simulink model "case8"  (R2024b)
settings: Solver=FixedStepAuto  StartTime=0  StopTime=1  FixedStep=1e-7  RelTol=1e-3
values from neighbouring files (symbols this model uses):
  SG_D_1_D = 0.01056    [IEEE9_case_parameters.m]    (also in case1_parameters.m; case2_parameters.m; case3_parameters.m; case4_parameters.m)
  SG_D_1_EnableSaturation = 0    [IEEE9_case_parameters.m]    (also in case1_parameters.m; case2_parameters.m; case3_parameters.m; case4_parameters.m)
  SG_D_1_f0 = 60    [IEEE9_case_parameters.m]    (also in case1_parameters.m; case2_parameters.m; case3_parameters.m; case4_parameters.m)
  SG_D_1_H = 7.5    [IEEE9_case_parameters.m]    (also in case1_parameters.m; case2_parameters.m; case3_parameters.m; case4_parameters.m)
  SG_D_1_K_A = 20    [IEEE9_case_parameters.m]    (also in case1_parameters.m; case2_parameters.m; case3_parameters.m; case4_parameters.m)
  SG_D_1_K_E = 1.000000e+1    (= 10)    [IEEE9_case_parameters.m]    (also in case1_parameters.m; case2_parameters.m; case3_parameters.m; case4_parameters.m)
  SG_D_1_K_F = 2.363    [IEEE9_case_parameters.m]    (also in case1_parameters.m; case2_parameters.m; case3_parameters.m; case4_parameters.m)
  SG_D_1_K_s = 0.5    [IEEE9_case_parameters.m]    (also in case1_parameters.m = 5; case2_parameters.m = 5; case3_parameters.m = 5; case4_parameters.m = 5)
  SG_D_1_R_a = 0.001088    [IEEE9_case_parameters.m]    (also in case1_parameters.m; case2_parameters.m; case3_parameters.m; case4_parameters.m)
  SG_D_1_S_A = 1    [IEEE9_case_parameters.m]    (also in case1_parameters.m; case2_parameters.m; case3_parameters.m; case4_parameters.m)
  SG_D_1_S_B = 0.103    [IEEE9_case_parameters.m]    (also in case1_parameters.m; case2_parameters.m; case3_parameters.m; case4_parameters.m)
  SG_D_1_S_N = 10.659857    [IEEE9_case_parameters.m]    (also in case1_parameters.m; case2_parameters.m; case3_parameters.m; case4_parameters.m)
  SG_D_1_SpeedPara = 200    [IEEE9_case_parameters.m]    (also in case1_parameters.m; case2_parameters.m; case3_parameters.m; case4_parameters.m)
  SG_D_1_T_0 = 0.720173    [IEEE9_case_parameters.m]    (also in case1_parameters.m = 0.755522; case2_parameters.m = 0.808931; case3_parameters.m = 0.869402; case4_parameters.m = 0.729316)
  SG_D_1_T_1 = 0.3    [IEEE9_case_parameters.m]    (also in case1_parameters.m; case2_parameters.m; case3_parameters.m; case4_parameters.m)
  SG_D_1_T_2 = 0.05    [IEEE9_case_parameters.m]    (also in case1_parameters.m; case2_parameters.m; case3_parameters.m; case4_parameters.m)
  SG_D_1_T_3 = 0.02    [IEEE9_case_parameters.m]    (also in case1_parameters.m; case2_parameters.m; case3_parameters.m; case4_parameters.m)
  SG_D_1_T_4 = 0.005    [IEEE9_case_parameters.m]    (also in case1_parameters.m; case2_parameters.m; case3_parameters.m; case4_parameters.m)
  SG_D_1_T_A = 0.02    [IEEE9_case_parameters.m]    (also in case1_parameters.m; case2_parameters.m; case3_parameters.m; case4_parameters.m)
  SG_D_1_T_dd = 8.000000e+0    (= 8)    [IEEE9_case_parameters.m]    (also in case1_parameters.m; case2_parameters.m; case3_parameters.m; case4_parameters.m)
  SG_D_1_T_ddd = 0.04    [IEEE9_case_parameters.m]    (also in case1_parameters.m; case2_parameters.m; case3_parameters.m; case4_parameters.m)
  SG_D_1_T_E = 0.314    [IEEE9_case_parameters.m]    (also in case1_parameters.m; case2_parameters.m; case3_parameters.m; case4_parameters.m)
  SG_D_1_T_F = 0.35    [IEEE9_case_parameters.m]    (also in case1_parameters.m; case2_parameters.m; case3_parameters.m; case4_parameters.m)
  SG_D_1_T_qd = 0.8    [IEEE9_case_parameters.m]    (also in case1_parameters.m; case2_parameters.m; case3_parameters.m; case4_parameters.m)
  SG_D_1_T_qdd = 0.02    [IEEE9_case_parameters.m]    (also in case1_parameters.m; case2_parameters.m; case3_parameters.m; case4_parameters.m)
  SG_D_1_T_speed = 0.1    [IEEE9_case_parameters.m]    (also in case1_parameters.m = 200; case2_parameters.m = 200; case3_parameters.m = 200; case4_parameters.m = 200)
  SG_D_1_T_w = 0.5    [IEEE9_case_parameters.m]    (also in case1_parameters.m; case2_parameters.m; case3_parameters.m; case4_parameters.m)
  SG_D_1_V_ref = 1.990276    [IEEE9_case_parameters.m]    (also in case1_parameters.m = 2.042296; case2_parameters.m = 2.051388; case3_parameters.m = 2.089584; case4_parameters.m = 2.01845)
  SG_D_1_w_ref = 376.991118    [IEEE9_case_parameters.m]    (also in case1_parameters.m; case2_parameters.m; case3_parameters.m; case4_parameters.m)
  SG_D_1_wb = 6.000000e+1    (= 60)    [IEEE9_case_parameters.m]    (also in case1_parameters.m; case2_parameters.m; case3_parameters.m; case4_parameters.m)
  SG_D_1_x_d = 1.9    [IEEE9_case_parameters.m]    (also in case1_parameters.m; case2_parameters.m; case3_parameters.m; case4_parameters.m)
  SG_D_1_x_dd = 0.302    [IEEE9_case_parameters.m]    (also in case1_parameters.m; case2_parameters.m; case3_parameters.m; case4_parameters.m)
  SG_D_1_x_ddd = 0.204    [IEEE9_case_parameters.m]    (also in case1_parameters.m; case2_parameters.m; case3_parameters.m; case4_parameters.m)
  SG_D_1_x_l = 0.05    [IEEE9_case_parameters.m]    (also in case1_parameters.m; case2_parameters.m; case3_parameters.m; case4_parameters.m)
  SG_D_1_x_q = 1.3    [IEEE9_case_parameters.m]    (also in case1_parameters.m; case2_parameters.m; case3_parameters.m; case4_parameters.m)
  SG_D_1_x_qd = 0.5    [IEEE9_case_parameters.m]    (also in case1_parameters.m; case2_parameters.m; case3_parameters.m; case4_parameters.m)
  SG_D_1_x_qdd = 0.3    [IEEE9_case_parameters.m]    (also in case1_parameters.m; case2_parameters.m; case3_parameters.m; case4_parameters.m)
  SG_D_2_D = 0.02    [IEEE9_case_parameters.m]    (also in case1_parameters.m; case2_parameters.m; case3_parameters.m; case4_parameters.m)
  SG_D_2_EnableSaturation = 0    [IEEE9_case_parameters.m]    (also in case1_parameters.m; case2_parameters.m; case3_parameters.m; case4_parameters.m)
  SG_D_2_f0 = 60    [IEEE9_case_parameters.m]    (also in case1_parameters.m; case2_parameters.m; case3_parameters.m; case4_parameters.m)
  SG_D_2_H = 8.000000e+0    (= 8)    [IEEE9_case_parameters.m]    (also in case1_parameters.m; case2_parameters.m; case3_parameters.m; case4_parameters.m)
  SG_D_2_K_A = 20    [IEEE9_case_parameters.m]    (also in case1_parameters.m; case2_parameters.m; case3_parameters.m; case4_parameters.m)
  SG_D_2_K_E = 1.000000e+1    (= 10)    [IEEE9_case_parameters.m]    (also in case1_parameters.m; case2_parameters.m; case3_parameters.m; case4_parameters.m)
  SG_D_2_K_F = 2.363    [IEEE9_case_parameters.m]    (also in case1_parameters.m; case2_parameters.m; case3_parameters.m; case4_parameters.m)
  SG_D_2_K_s = 0.5    [IEEE9_case_parameters.m]    (also in case1_parameters.m = 4; case2_parameters.m = 4; case3_parameters.m = 4; case4_parameters.m = 4)
  SG_D_2_R_a = 0.001088    [IEEE9_case_parameters.m]    (also in case1_parameters.m; case2_parameters.m; case3_parameters.m; case4_parameters.m)
  SG_D_2_S_A = 1    [IEEE9_case_parameters.m]    (also in case1_parameters.m; case2_parameters.m; case3_parameters.m; case4_parameters.m)
  SG_D_2_S_B = 0.103    [IEEE9_case_parameters.m]    (also in case1_parameters.m; case2_parameters.m; case3_parameters.m; case4_parameters.m)
  SG_D_2_S_N = 10.659857    [IEEE9_case_parameters.m]    (also in case1_parameters.m; case2_parameters.m; case3_parameters.m; case4_parameters.m)
  SG_D_2_SpeedPara = 200    [IEEE9_case_parameters.m]    (also in case1_parameters.m; case2_parameters.m; case3_parameters.m; case4_parameters.m)
  SG_D_2_T_0 = 1.632913    [IEEE9_case_parameters.m]    (also in case1_parameters.m = 1.632925; case2_parameters.m = 1.632915; case3_parameters.m = 1.632914; case4_parameters.m = 1.632927)
  SG_D_2_T_1 = 0.2    [IEEE9_case_parameters.m]    (also in case1_parameters.m; case2_parameters.m; case3_parameters.m; case4_parameters.m)
  SG_D_2_T_2 = 0.05    [IEEE9_case_parameters.m]    (also in case1_parameters.m; case2_parameters.m; case3_parameters.m; case4_parameters.m)
  SG_D_2_T_3 = 0.02    [IEEE9_case_parameters.m]    (also in case1_parameters.m; case2_parameters.m; case3_parameters.m; case4_parameters.m)
  SG_D_2_T_4 = 0.005    [IEEE9_case_parameters.m]    (also in case1_parameters.m; case2_parameters.m; case3_parameters.m; case4_parameters.m)
  SG_D_2_T_A = 0.02    [IEEE9_case_parameters.m]    (also in case1_parameters.m; case2_parameters.m; case3_parameters.m; case4_parameters.m)
  SG_D_2_T_dd = 7.9    [IEEE9_case_parameters.m]    (also in case1_parameters.m; case2_parameters.m; case3_parameters.m; case4_parameters.m)
  SG_D_2_T_ddd = 0.04    [IEEE9_case_parameters.m]    (also in case1_parameters.m; case2_parameters.m; case3_parameters.m; case4_parameters.m)
  SG_D_2_T_E = 0.314    [IEEE9_case_parameters.m]    (also in case1_parameters.m; case2_parameters.m; case3_parameters.m; case4_parameters.m)
  SG_D_2_T_F = 0.35    [IEEE9_case_parameters.m]    (also in case1_parameters.m; case2_parameters.m; case3_parameters.m; case4_parameters.m)
  SG_D_2_T_qd = 0.8    [IEEE9_case_parameters.m]    (also in case1_parameters.m; case2_parameters.m; case3_parameters.m; case4_parameters.m)
  SG_D_2_T_qdd = 0.015    [IEEE9_case_parameters.m]    (also in case1_parameters.m; case2_parameters.m; case3_parameters.m; case4_parameters.m)
  SG_D_2_T_speed = 0.1    [IEEE9_case_parameters.m]    (also in case1_parameters.m = 150; case2_parameters.m = 150; case3_parameters.m = 150; case4_parameters.m = 150)
  SG_D_2_T_w = 0.35    [IEEE9_case_parameters.m]    (also in case1_parameters.m; case2_parameters.m; case3_parameters.m; case4_parameters.m)
  SG_D_2_V_ref = 2.58547    [IEEE9_case_parameters.m]    (also in case1_parameters.m = 2.597896; case2_parameters.m = 2.587136; case3_parameters.m = 2.586042; case4_parameters.m = 2.599679)
  SG_D_2_w_ref = 376.991118    [IEEE9_case_parameters.m]    (also in case1_parameters.m; case2_parameters.m; case3_parameters.m; case4_parameters.m)
  SG_D_2_wb = 6.000000e+1    (= 60)    [IEEE9_case_parameters.m]    (also in case1_parameters.m; case2_parameters.m; case3_parameters.m; case4_parameters.m)
  SG_D_2_x_d = 1.8    [IEEE9_case_parameters.m]    (also in case1_parameters.m; case2_parameters.m; case3_parameters.m; case4_parameters.m)
  SG_D_2_x_dd = 0.302    [IEEE9_case_parameters.m]    (also in case1_parameters.m; case2_parameters.m; case3_parameters.m; case4_parameters.m)
  SG_D_2_x_ddd = 0.204    [IEEE9_case_parameters.m]    (also in case1_parameters.m; case2_parameters.m; case3_parameters.m; case4_parameters.m)
  SG_D_2_x_l = 0.05    [IEEE9_case_parameters.m]    (also in case1_parameters.m; case2_parameters.m; case3_parameters.m; case4_parameters.m)
  SG_D_2_x_q = 1.25    [IEEE9_case_parameters.m]    (also in case1_parameters.m; case2_parameters.m; case3_parameters.m; case4_parameters.m)
  SG_D_2_x_qd = 0.5    [IEEE9_case_parameters.m]    (also in case1_parameters.m; case2_parameters.m; case3_parameters.m; case4_parameters.m)
  SG_D_2_x_qdd = 0.3    [IEEE9_case_parameters.m]    (also in case1_parameters.m; case2_parameters.m; case3_parameters.m; case4_parameters.m)
  SG_D_3_D = 0.02    [IEEE9_case_parameters.m]    (also in case1_parameters.m; case2_parameters.m; case3_parameters.m; case4_parameters.m)
  SG_D_3_EnableSaturation = 0    [IEEE9_case_parameters.m]    (also in case1_parameters.m; case2_parameters.m; case3_parameters.m; case4_parameters.m)
  SG_D_3_f0 = 60    [IEEE9_case_parameters.m]    (also in case1_parameters.m; case2_parameters.m; case3_parameters.m; case4_parameters.m)
  SG_D_3_H = 7.7    [IEEE9_case_parameters.m]    (also in case1_parameters.m; case2_parameters.m; case3_parameters.m; case4_parameters.m)
  SG_D_3_K_A = 20    [IEEE9_case_parameters.m]    (also in case1_parameters.m; case2_parameters.m; case3_parameters.m; case4_parameters.m)
  SG_D_3_K_E = 1.000000e+1    (= 10)    [IEEE9_case_parameters.m]    (also in case1_parameters.m; case2_parameters.m; case3_parameters.m; case4_parameters.m)
  SG_D_3_K_F = 2.363    [IEEE9_case_parameters.m]    (also in case1_parameters.m; case2_parameters.m; case3_parameters.m; case4_parameters.m)
  SG_D_3_K_s = 0.2    [IEEE9_case_parameters.m]    (also in case1_parameters.m = 2; case2_parameters.m = 2; case3_parameters.m = 2; case4_parameters.m = 2)
  SG_D_3_R_a = 0.001088    [IEEE9_case_parameters.m]    (also in case1_parameters.m; case2_parameters.m; case3_parameters.m; case4_parameters.m)
  SG_D_3_S_A = 1    [IEEE9_case_parameters.m]    (also in case1_parameters.m; case2_parameters.m; case3_parameters.m; case4_parameters.m)
  SG_D_3_S_B = 0.103    [IEEE9_case_parameters.m]    (also in case1_parameters.m; case2_parameters.m; case3_parameters.m; case4_parameters.m)
  SG_D_3_S_N = 10.659857    [IEEE9_case_parameters.m]    (also in case1_parameters.m; case2_parameters.m; case3_parameters.m; case4_parameters.m)
  SG_D_3_SpeedPara = 200    [IEEE9_case_parameters.m]    (also in case1_parameters.m; case2_parameters.m; case3_parameters.m; case4_parameters.m)
  SG_D_3_T_0 = 0.850788    [IEEE9_case_parameters.m]    (also in case1_parameters.m = 0.850786; case2_parameters.m = 0.850787; case3_parameters.m; case4_parameters.m = 0.850786)
  SG_D_3_T_1 = 0.2    [IEEE9_case_parameters.m]    (also in case1_parameters.m; case2_parameters.m; case3_parameters.m; case4_parameters.m)
  SG_D_3_T_2 = 0.05    [IEEE9_case_parameters.m]    (also in case1_parameters.m; case2_parameters.m; case3_parameters.m; case4_parameters.m)
  SG_D_3_T_3 = 0.02    [IEEE9_case_parameters.m]    (also in case1_parameters.m; case2_parameters.m; case3_parameters.m; case4_parameters.m)
  SG_D_3_T_4 = 0.005    [IEEE9_case_parameters.m]    (also in case1_parameters.m; case2_parameters.m; case3_parameters.m; case4_parameters.m)
  SG_D_3_T_A = 0.02    [IEEE9_case_parameters.m]    (also in case1_parameters.m; case2_parameters.m; case3_parameters.m; case4_parameters.m)
  SG_D_3_T_dd = 8.1    [IEEE9_case_parameters.m]    (also in case1_parameters.m; case2_parameters.m; case3_parameters.m; case4_parameters.m)
  SG_D_3_T_ddd = 0.04    [IEEE9_case_parameters.m]    (also in case1_parameters.m; case2_parameters.m; case3_parameters.m; case4_parameters.m)
  SG_D_3_T_E = 0.314    [IEEE9_case_parameters.m]    (also in case1_parameters.m; case2_parameters.m; case3_parameters.m; case4_parameters.m)
  SG_D_3_T_F = 0.35    [IEEE9_case_parameters.m]    (also in case1_parameters.m; case2_parameters.m; case3_parameters.m; case4_parameters.m)
  SG_D_3_T_qd = 0.8    [IEEE9_case_parameters.m]    (also in case1_parameters.m; case2_parameters.m; case3_parameters.m; case4_parameters.m)
  SG_D_3_T_qdd = 0.015    [IEEE9_case_parameters.m]    (also in case1_parameters.m; case2_parameters.m; case3_parameters.m; case4_parameters.m)
  SG_D_3_T_speed = 0.1    [IEEE9_case_parameters.m]    (also in case1_parameters.m = 180; case2_parameters.m = 180; case3_parameters.m = 180; case4_parameters.m = 180)
  SG_D_3_T_w = 0.4    [IEEE9_case_parameters.m]    (also in case1_parameters.m; case2_parameters.m; case3_parameters.m; case4_parameters.m)
  SG_D_3_V_ref = 1.892727    [IEEE9_case_parameters.m]    (also in case1_parameters.m = 1.906439; case2_parameters.m = 1.895535; case3_parameters.m = 1.892105; case4_parameters.m = 1.906598)
  SG_D_3_w_ref = 376.991118    [IEEE9_case_parameters.m]    (also in case1_parameters.m; case2_parameters.m; case3_parameters.m; case4_parameters.m)
  SG_D_3_wb = 6.000000e+1    (= 60)    [IEEE9_case_parameters.m]    (also in case1_parameters.m; case2_parameters.m; case3_parameters.m; case4_parameters.m)
  SG_D_3_x_d = 1.85    [IEEE9_case_parameters.m]    (also in case1_parameters.m; case2_parameters.m; case3_parameters.m; case4_parameters.m)
  SG_D_3_x_dd = 0.302    [IEEE9_case_parameters.m]    (also in case1_parameters.m; case2_parameters.m; case3_parameters.m; case4_parameters.m)
  SG_D_3_x_ddd = 0.204    [IEEE9_case_parameters.m]    (also in case1_parameters.m; case2_parameters.m; case3_parameters.m; case4_parameters.m)
  SG_D_3_x_l = 0.05    [IEEE9_case_parameters.m]    (also in case1_parameters.m; case2_parameters.m; case3_parameters.m; case4_parameters.m)
  SG_D_3_x_q = 1.2    [IEEE9_case_parameters.m]    (also in case1_parameters.m; case2_parameters.m; case3_parameters.m; case4_parameters.m)
  SG_D_3_x_qd = 0.5    [IEEE9_case_parameters.m]    (also in case1_parameters.m; case2_parameters.m; case3_parameters.m; case4_parameters.m)
  SG_D_3_x_qdd = 0.3    [IEEE9_case_parameters.m]    (also in case1_parameters.m; case2_parameters.m; case3_parameters.m; case4_parameters.m)
(part 4 of 12)

== system case8/AC_1/d_vq_bus_7_block ==
  note: d_vq_bus_7 in case8
      | $2106.09563369148\,\mathrm{iq}_{\mathrm{bus},7}-376.991118430775\,\mathrm{vd}_{\mathrm{bus},7}$
      | Automatically generated on 2025-10-31 19:30:28 .
  Alge_iq_bus_7_726e3 : Inport
  State_vd_bus_7_2248a : Inport  Port=2
  Constant_2106.09563369148_b3474 : Constant  Value=2106.09563369148
  Constant_376.991118430775_43736 : Constant  Value=376.991118430775
  Product_03bd9 : Product
  Product_7ad7e : Product
  Subtract_cbf81 : Sum  Inputs=+-
  Blockout_d_vq_bus_7_abefa : Outport
  wires:
  Constant_2106.09563369148_b3474/1 -> Product_03bd9/1
  Product_7ad7e/1 -> Subtract_cbf81/2
  Alge_iq_bus_7_726e3/1 -> Product_03bd9/2
  Constant_376.991118430775_43736/1 -> Product_7ad7e/1
  Subtract_cbf81/1 -> Blockout_d_vq_bus_7_abefa/1
  State_vd_bus_7_2248a/1 -> Product_7ad7e/2
  Product_03bd9/1 -> Subtract_cbf81/1

== system case8/AC_1/d_vq_bus_8_block ==
  note: d_vq_bus_8 in case8
      | $1657.10381727813\,\mathrm{iq}_{\mathrm{bus},8}-376.991118430775\,\mathrm{vd}_{\mathrm{bus},8}$
      | Automatically generated on 2025-10-31 19:30:28 .
  Alge_iq_bus_8_62ae5 : Inport
  State_vd_bus_8_5f7c7 : Inport  Port=2
  Constant_1657.10381727813_c6206 : Constant  Value=1657.10381727813
  Constant_376.991118430775_d5aa6 : Constant  Value=376.991118430775
  Product_11353 : Product
  Product_98297 : Product
  Subtract_bf7b5 : Sum  Inputs=+-
  Blockout_d_vq_bus_8_a6a13 : Outport
  wires:
  Constant_1657.10381727813_c6206/1 -> Product_11353/1
  Constant_376.991118430775_d5aa6/1 -> Product_98297/1
  Alge_iq_bus_8_62ae5/1 -> Product_11353/2
  State_vd_bus_8_5f7c7/1 -> Product_98297/2
  Product_11353/1 -> Subtract_bf7b5/1
  Product_98297/1 -> Subtract_bf7b5/2
  Subtract_bf7b5/1 -> Blockout_d_vq_bus_8_a6a13/1

== system case8/AC_1/d_vq_bus_9_block ==
  note: d_vq_bus_9 in case8
      | $1564.27849971276\,\mathrm{iq}_{\mathrm{bus},9}-376.991118430775\,\mathrm{vd}_{\mathrm{bus},9}$
      | Automatically generated on 2025-10-31 19:30:29 .
  Alge_iq_bus_9_567ad : Inport
  State_vd_bus_9_b5567 : Inport  Port=2
  Constant_1564.27849971276_965ff : Constant  Value=1564.27849971276
  Constant_376.991118430775_88cbd : Constant  Value=376.991118430775
  Product_85d09 : Product
  Product_ef330 : Product
  Subtract_a67ef : Sum  Inputs=+-
  Blockout_d_vq_bus_9_8c5c4 : Outport
  wires:
  Constant_1564.27849971276_965ff/1 -> Product_85d09/1
  Constant_376.991118430775_88cbd/1 -> Product_ef330/1
  Alge_iq_bus_9_567ad/1 -> Product_85d09/2
  State_vd_bus_9_b5567/1 -> Product_ef330/2
  Product_85d09/1 -> Subtract_a67ef/1
  Product_ef330/1 -> Subtract_a67ef/2
  Subtract_a67ef/1 -> Blockout_d_vq_bus_9_8c5c4/1

== system case8/AC_1/id_bus_1_block ==
  note: id_bus_1 in case8
      | $\mathrm{id}_{\mathrm{SG},D,1}-\mathrm{id}_{\mathrm{line},1,4}$
      | Automatically generated on 2025-10-31 19:30:39 .
  Input_id_SG_D_1_34d26 : Inport
  State_id_line_1_4_fde27 : Inport  Port=2
  Subtract_d19f4 : Sum  Inputs=+-
  Blockout_id_bus_1_cb042 : Outport
  wires:
  Input_id_SG_D_1_34d26/1 -> Subtract_d19f4/1
  State_id_line_1_4_fde27/1 -> Subtract_d19f4/2
  Subtract_d19f4/1 -> Blockout_id_bus_1_cb042/1

== system case8/AC_1/id_bus_2_block ==
  note: id_bus_2 in case8
      | $\mathrm{id}_{\mathrm{SG},D,2}+\mathrm{id}_{\mathrm{line},8,2}$
      | Automatically generated on 2025-10-31 19:30:40 .
  Input_id_SG_D_2_c44ab : Inport
  State_id_line_8_2_faf95 : Inport  Port=2
  Add_08d47 : Sum
  Blockout_id_bus_2_80de6 : Outport
  wires:
  Input_id_SG_D_2_c44ab/1 -> Add_08d47/1
  State_id_line_8_2_faf95/1 -> Add_08d47/2
  Add_08d47/1 -> Blockout_id_bus_2_80de6/1

== system case8/AC_1/id_bus_3_block ==
  note: id_bus_3 in case8
      | $\mathrm{id}_{\mathrm{SG},D,3}-\mathrm{id}_{\mathrm{line},3,6}$
      | Automatically generated on 2025-10-31 19:30:41 .
  Input_id_SG_D_3_f75b7 : Inport
  State_id_line_3_6_5f9cc : Inport  Port=2
  Subtract_74bab : Sum  Inputs=+-
  Blockout_id_bus_3_50cd8 : Outport
  wires:
  Input_id_SG_D_3_f75b7/1 -> Subtract_74bab/1
  State_id_line_3_6_5f9cc/1 -> Subtract_74bab/2
  Subtract_74bab/1 -> Blockout_id_bus_3_50cd8/1

== system case8/AC_1/id_bus_4_block ==
  note: id_bus_4 in case8
      | $\mathrm{id}_{\mathrm{line},1,4}-\mathrm{id}_{\mathrm{line},4,5}+\mathrm{id}_{\mathrm{line},9,4}$
      | Automatically generated on 2025-10-31 19:30:41 .
  State_id_line_1_4_affcb : Inport
  State_id_line_4_5_51819 : Inport  Port=2
  State_id_line_9_4_afd85 : Inport  Port=3
  Add_37faf : Sum
  Subtract_9fc5a : Sum  Inputs=+-
  Blockout_id_bus_4_7de9e : Outport
  wires:
  State_id_line_9_4_afd85/1 -> Add_37faf/2
  State_id_line_1_4_affcb/1 -> Subtract_9fc5a/1
  State_id_line_4_5_51819/1 -> Subtract_9fc5a/2
  Subtract_9fc5a/1 -> Add_37faf/1
  Add_37faf/1 -> Blockout_id_bus_4_7de9e/1

== system case8/AC_1/id_bus_5_block ==
  note: id_bus_5 in case8
      | $\mathrm{id}_{\mathrm{line},4,5}-\mathrm{id}_{\mathrm{load},5}-\mathrm{id}_{\mathrm{line},5,6}$
      | Automatically generated on 2025-10-31 19:30:42 .
  State_id_load_5_a095c : Inport
  State_id_line_4_5_ebaf3 : Inport  Port=2
  State_id_line_5_6_9ddb2 : Inport  Port=3
  Add_54ae7 : Sum
  Constant_-1_b8b63 : Constant  Value=-1
  Product_79816 : Product
  Subtract_84ece : Sum  Inputs=+-
  Blockout_id_bus_5_cac9d : Outport
  wires:
  Subtract_84ece/1 -> Blockout_id_bus_5_cac9d/1
  State_id_line_4_5_ebaf3/1 -> Add_54ae7/2
  Constant_-1_b8b63/1 -> Product_79816/1
  Add_54ae7/1 -> Subtract_84ece/1
  State_id_load_5_a095c/1 -> Product_79816/2
  Product_79816/1 -> Add_54ae7/1
  State_id_line_5_6_9ddb2/1 -> Subtract_84ece/2

== system case8/AC_1/id_bus_6_block ==
  note: id_bus_6 in case8
      | $\mathrm{id}_{\mathrm{line},3,6}+\mathrm{id}_{\mathrm{line},5,6}-\mathrm{id}_{\mathrm{line},6,7}$
      | Automatically generated on 2025-10-31 19:30:42 .
  State_id_line_3_6_f75bf : Inport
  State_id_line_5_6_dde6e : Inport  Port=2
  State_id_line_6_7_7cee2 : Inport  Port=3
  Add_2188b : Sum
  Subtract_f5ef8 : Sum  Inputs=+-
  Blockout_id_bus_6_83936 : Outport
  wires:
  State_id_line_6_7_7cee2/1 -> Subtract_f5ef8/2
  State_id_line_3_6_f75bf/1 -> Add_2188b/1
  State_id_line_5_6_dde6e/1 -> Add_2188b/2
  Add_2188b/1 -> Subtract_f5ef8/1
  Subtract_f5ef8/1 -> Blockout_id_bus_6_83936/1

== system case8/AC_1/id_bus_7_block ==
  note: id_bus_7 in case8
      | $\mathrm{id}_{\mathrm{line},6,7}-\mathrm{id}_{\mathrm{load},7}-\mathrm{id}_{\mathrm{line},7,8}$
      | Automatically generated on 2025-10-31 19:30:43 .
  State_id_load_7_ee538 : Inport
  State_id_line_6_7_45ba3 : Inport  Port=2
  State_id_line_7_8_7eef9 : Inport  Port=3
  Add_5909c : Sum
  Constant_-1_723c1 : Constant  Value=-1
  Product_3f30b : Product
  Subtract_ba02b : Sum  Inputs=+-
  Blockout_id_bus_7_7ae2c : Outport
  wires:
  Subtract_ba02b/1 -> Blockout_id_bus_7_7ae2c/1
  State_id_line_6_7_45ba3/1 -> Add_5909c/2
  Constant_-1_723c1/1 -> Product_3f30b/1
  Add_5909c/1 -> Subtract_ba02b/1
  State_id_load_7_ee538/1 -> Product_3f30b/2
  Product_3f30b/1 -> Add_5909c/1
  State_id_line_7_8_7eef9/1 -> Subtract_ba02b/2

== system case8/AC_1/id_bus_8_block ==
  note: id_bus_8 in case8
      | $\mathrm{id}_{\mathrm{line},7,8}-\mathrm{id}_{\mathrm{line},8,2}-\mathrm{id}_{\mathrm{line},8,9}$
      | Automatically generated on 2025-10-31 19:30:43 .
  State_id_line_7_8_15e81 : Inport
  State_id_line_8_2_77f88 : Inport  Port=2
  State_id_line_8_9_98e94 : Inport  Port=3
  Subtract_11052 : Sum  Inputs=+-
  Subtract_3f731 : Sum  Inputs=+-
  Blockout_id_bus_8_70ccf : Outport
  wires:
  State_id_line_8_9_98e94/1 -> Subtract_3f731/2
  State_id_line_7_8_15e81/1 -> Subtract_11052/1
  State_id_line_8_2_77f88/1 -> Subtract_11052/2
  Subtract_11052/1 -> Subtract_3f731/1
  Subtract_3f731/1 -> Blockout_id_bus_8_70ccf/1

== system case8/AC_1/id_bus_9_block ==
  note: id_bus_9 in case8
      | $\mathrm{id}_{\mathrm{line},8,9}-\mathrm{id}_{\mathrm{load},9}-\mathrm{id}_{\mathrm{line},9,4}$
      | Automatically generated on 2025-10-31 19:30:44 .
  State_id_load_9_a44c9 : Inport
  State_id_line_8_9_50f90 : Inport  Port=2
  State_id_line_9_4_ac093 : Inport  Port=3
  Add_0df5a : Sum
  Constant_-1_15f7e : Constant  Value=-1
  Product_81357 : Product
  Subtract_c7e6c : Sum  Inputs=+-
  Blockout_id_bus_9_8caa0 : Outport
  wires:
  Subtract_c7e6c/1 -> Blockout_id_bus_9_8caa0/1
  State_id_line_8_9_50f90/1 -> Add_0df5a/2
  Constant_-1_15f7e/1 -> Product_81357/1
  Add_0df5a/1 -> Subtract_c7e6c/1
  State_id_load_9_a44c9/1 -> Product_81357/2
  Product_81357/1 -> Add_0df5a/1
  State_id_line_9_4_ac093/1 -> Subtract_c7e6c/2

== system case8/AC_1/iq_bus_1_block ==
  note: iq_bus_1 in case8
      | $\mathrm{iq}_{\mathrm{SG},D,1}-\mathrm{iq}_{\mathrm{line},1,4}$
      | Automatically generated on 2025-10-31 19:30:40 .
  Input_iq_SG_D_1_5d44b : Inport
  State_iq_line_1_4_1856f : Inport  Port=2
  Subtract_f0aa3 : Sum  Inputs=+-
  Blockout_iq_bus_1_b5acd : Outport
  wires:
  Input_iq_SG_D_1_5d44b/1 -> Subtract_f0aa3/1
  State_iq_line_1_4_1856f/1 -> Subtract_f0aa3/2
  Subtract_f0aa3/1 -> Blockout_iq_bus_1_b5acd/1

== system case8/AC_1/iq_bus_2_block ==
  note: iq_bus_2 in case8
      | $\mathrm{iq}_{\mathrm{SG},D,2}+\mathrm{iq}_{\mathrm{line},8,2}$
      | Automatically generated on 2025-10-31 19:30:40 .
  Input_iq_SG_D_2_5a31b : Inport
  State_iq_line_8_2_29be9 : Inport  Port=2
  Add_e80c5 : Sum
  Blockout_iq_bus_2_4440e : Outport
  wires:
  Input_iq_SG_D_2_5a31b/1 -> Add_e80c5/1
  State_iq_line_8_2_29be9/1 -> Add_e80c5/2
  Add_e80c5/1 -> Blockout_iq_bus_2_4440e/1

== system case8/AC_1/iq_bus_3_block ==
  note: iq_bus_3 in case8
      | $\mathrm{iq}_{\mathrm{SG},D,3}-\mathrm{iq}_{\mathrm{line},3,6}$
      | Automatically generated on 2025-10-31 19:30:41 .
  Input_iq_SG_D_3_5d10c : Inport
  State_iq_line_3_6_5365a : Inport  Port=2
  Subtract_671dd : Sum  Inputs=+-
  Blockout_iq_bus_3_1a2d8 : Outport
  wires:
  Input_iq_SG_D_3_5d10c/1 -> Subtract_671dd/1
  State_iq_line_3_6_5365a/1 -> Subtract_671dd/2
  Subtract_671dd/1 -> Blockout_iq_bus_3_1a2d8/1

== system case8/AC_1/iq_bus_4_block ==
  note: iq_bus_4 in case8
      | $\mathrm{iq}_{\mathrm{line},1,4}-\mathrm{iq}_{\mathrm{line},4,5}+\mathrm{iq}_{\mathrm{line},9,4}$
      | Automatically generated on 2025-10-31 19:30:42 .
  State_iq_line_1_4_e84c9 : Inport
  State_iq_line_4_5_3660f : Inport  Port=2
  State_iq_line_9_4_fec9c : Inport  Port=3
  Add_26994 : Sum
  Subtract_6a700 : Sum  Inputs=+-
  Blockout_iq_bus_4_34493 : Outport
  wires:
  State_iq_line_1_4_e84c9/1 -> Subtract_6a700/1
  State_iq_line_4_5_3660f/1 -> Subtract_6a700/2
  Subtract_6a700/1 -> Add_26994/1
  State_iq_line_9_4_fec9c/1 -> Add_26994/2
  Add_26994/1 -> Blockout_iq_bus_4_34493/1

== system case8/AC_1/iq_bus_5_block ==
  note: iq_bus_5 in case8
      | $\mathrm{iq}_{\mathrm{line},4,5}-\mathrm{iq}_{\mathrm{load},5}-\mathrm{iq}_{\mathrm{line},5,6}$
      | Automatically generated on 2025-10-31 19:30:42 .
  State_iq_load_5_7347c : Inport
  State_iq_line_4_5_0123c : Inport  Port=2
  State_iq_line_5_6_34d88 : Inport  Port=3
  Add_9b6a5 : Sum
  Constant_-1_ee194 : Constant  Value=-1
  Product_88b6f : Product
  Subtract_c3a79 : Sum  Inputs=+-
  Blockout_iq_bus_5_2f438 : Outport
  wires:
  Subtract_c3a79/1 -> Blockout_iq_bus_5_2f438/1
  State_iq_line_4_5_0123c/1 -> Add_9b6a5/2
  Constant_-1_ee194/1 -> Product_88b6f/1
  State_iq_load_5_7347c/1 -> Product_88b6f/2
  Product_88b6f/1 -> Add_9b6a5/1
  Add_9b6a5/1 -> Subtract_c3a79/1
  State_iq_line_5_6_34d88/1 -> Subtract_c3a79/2

== system case8/AC_1/iq_bus_6_block ==
  note: iq_bus_6 in case8
      | $\mathrm{iq}_{\mathrm{line},3,6}+\mathrm{iq}_{\mathrm{line},5,6}-\mathrm{iq}_{\mathrm{line},6,7}$
      | Automatically generated on 2025-10-31 19:30:43 .
  State_iq_line_3_6_d82ab : Inport
  State_iq_line_5_6_a2b8b : Inport  Port=2
  State_iq_line_6_7_6c502 : Inport  Port=3
  Add_5de9e : Sum
  Subtract_db680 : Sum  Inputs=+-
  Blockout_iq_bus_6_da1e9 : Outport
  wires:
  State_iq_line_3_6_d82ab/1 -> Add_5de9e/1
  State_iq_line_5_6_a2b8b/1 -> Add_5de9e/2
  Add_5de9e/1 -> Subtract_db680/1
  State_iq_line_6_7_6c502/1 -> Subtract_db680/2
  Subtract_db680/1 -> Blockout_iq_bus_6_da1e9/1

== system case8/AC_1/iq_bus_7_block ==
  note: iq_bus_7 in case8
      | $\mathrm{iq}_{\mathrm{line},6,7}-\mathrm{iq}_{\mathrm{load},7}-\mathrm{iq}_{\mathrm{line},7,8}$
      | Automatically generated on 2025-10-31 19:30:43 .
  State_iq_load_7_8eba6 : Inport
  State_iq_line_6_7_5c1a2 : Inport  Port=2
  State_iq_line_7_8_dca19 : Inport  Port=3
  Add_aa1a3 : Sum
  Constant_-1_cd870 : Constant  Value=-1
  Product_ea23d : Product
  Subtract_593f2 : Sum  Inputs=+-
  Blockout_iq_bus_7_1d767 : Outport
  wires:
  Subtract_593f2/1 -> Blockout_iq_bus_7_1d767/1
  State_iq_line_6_7_5c1a2/1 -> Add_aa1a3/2
  Constant_-1_cd870/1 -> Product_ea23d/1
  State_iq_load_7_8eba6/1 -> Product_ea23d/2
  Product_ea23d/1 -> Add_aa1a3/1
  Add_aa1a3/1 -> Subtract_593f2/1
  State_iq_line_7_8_dca19/1 -> Subtract_593f2/2

== system case8/AC_1/iq_bus_8_block ==
  note: iq_bus_8 in case8
      | $\mathrm{iq}_{\mathrm{line},7,8}-\mathrm{iq}_{\mathrm{line},8,2}-\mathrm{iq}_{\mathrm{line},8,9}$
      | Automatically generated on 2025-10-31 19:30:44 .
  State_iq_line_7_8_8d26a : Inport
  State_iq_line_8_2_2aff1 : Inport  Port=2
  State_iq_line_8_9_c19e3 : Inport  Port=3
  Subtract_71d4c : Sum  Inputs=+-
  Subtract_78632 : Sum  Inputs=+-
  Blockout_iq_bus_8_09f70 : Outport
  wires:
  State_iq_line_7_8_8d26a/1 -> Subtract_71d4c/1
  State_iq_line_8_2_2aff1/1 -> Subtract_71d4c/2
  Subtract_71d4c/1 -> Subtract_78632/1
  State_iq_line_8_9_c19e3/1 -> Subtract_78632/2
  Subtract_78632/1 -> Blockout_iq_bus_8_09f70/1

== system case8/AC_1/iq_bus_9_block ==
  note: iq_bus_9 in case8
      | $\mathrm{iq}_{\mathrm{line},8,9}-\mathrm{iq}_{\mathrm{load},9}-\mathrm{iq}_{\mathrm{line},9,4}$
      | Automatically generated on 2025-10-31 19:30:44 .
  State_iq_load_9_87d2c : Inport
  State_iq_line_8_9_901dd : Inport  Port=2
  State_iq_line_9_4_3ae2e : Inport  Port=3
  Add_69340 : Sum
  Constant_-1_70571 : Constant  Value=-1
  Product_84eeb : Product
  Subtract_389ad : Sum  Inputs=+-
  Blockout_iq_bus_9_995fd : Outport
  wires:
  Subtract_389ad/1 -> Blockout_iq_bus_9_995fd/1
  State_iq_line_8_9_901dd/1 -> Add_69340/2
  Constant_-1_70571/1 -> Product_84eeb/1
  State_iq_load_9_87d2c/1 -> Product_84eeb/2
  Product_84eeb/1 -> Add_69340/1
  Add_69340/1 -> Subtract_389ad/1
  State_iq_line_9_4_3ae2e/1 -> Subtract_389ad/2

== system case8/AC_1/vd_bus_1_out_block ==
  note: vd_bus_1_out in case8
      | $\mathrm{vd}_{\mathrm{bus},1}$
      | Automatically generated on 2025-10-31 19:30:39 .
  State_vd_bus_1_c7201 : Inport
  Blockout_vd_bus_1_out_dd07e : Outport
  wires:
  State_vd_bus_1_c7201/1 -> Blockout_vd_bus_1_out_dd07e/1

== system case8/AC_1/vd_bus_2_out_block ==
  note: vd_bus_2_out in case8
      | $\mathrm{vd}_{\mathrm{bus},2}$
      | Automatically generated on 2025-10-31 19:30:40 .
  State_vd_bus_2_35c0c : Inport
  Blockout_vd_bus_2_out_2c03e : Outport
  wires:
  State_vd_bus_2_35c0c/1 -> Blockout_vd_bus_2_out_2c03e/1

== system case8/AC_1/vd_bus_3_out_block ==
  note: vd_bus_3_out in case8
      | $\mathrm{vd}_{\mathrm{bus},3}$
      | Automatically generated on 2025-10-31 19:30:41 .
  State_vd_bus_3_bb6c5 : Inport
  Blockout_vd_bus_3_out_b3a99 : Outport
  wires:
  State_vd_bus_3_bb6c5/1 -> Blockout_vd_bus_3_out_b3a99/1

== system case8/AC_1/vq_bus_1_out_block ==
  note: vq_bus_1_out in case8
      | $\mathrm{vq}_{\mathrm{bus},1}$
      | Automatically generated on 2025-10-31 19:30:39 .
  State_vq_bus_1_dbece : Inport
  Blockout_vq_bus_1_out_0bb6b : Outport
  wires:
  State_vq_bus_1_dbece/1 -> Blockout_vq_bus_1_out_0bb6b/1

== system case8/AC_1/vq_bus_2_out_block ==
  note: vq_bus_2_out in case8
      | $\mathrm{vq}_{\mathrm{bus},2}$
      | Automatically generated on 2025-10-31 19:30:40 .
  State_vq_bus_2_07eb1 : Inport
  Blockout_vq_bus_2_out_c20d3 : Outport
  wires:
  State_vq_bus_2_07eb1/1 -> Blockout_vq_bus_2_out_c20d3/1

== system case8/AC_1/vq_bus_3_out_block ==
  note: vq_bus_3_out in case8
      | $\mathrm{vq}_{\mathrm{bus},3}$
      | Automatically generated on 2025-10-31 19:30:41 .
  State_vq_bus_3_f0f91 : Inport
  Blockout_vq_bus_3_out_a7c8e : Outport
  wires:
  State_vq_bus_3_f0f91/1 -> Blockout_vq_bus_3_out_a7c8e/1

== system case8/SG_D_1/T_e_SG_D_1_block ==
  note: T_e_SG_D_1 in case8
      | $-\frac{\psi _{d,\mathrm{SG},D,1}\,\left(\psi _{q,\mathrm{SG},D,1}+\frac{\psi _{\mathrm{gq},\mathrm{SG},D,1}\,\left(x_{l}-x_{\mathrm{qdd}}\right)}{x_{l}-x_{\mathrm{qd}}}+\frac{\psi _{\mathrm{kq},\mathrm{SG},D,1}\,\left(x_{\mathrm{qd}}-x_{\mathrm{qdd}}\right)}{x_{l}-x_{\mathrm{qd}}}\right)}{x_{\mathrm{qdd}}}-\frac{\psi _{q,\mathrm{SG},D,1}\,\left(\frac{\psi _{\mathrm{1d},\mathrm{SG},D,1}\,\left(x_{\mathrm{dd}}-x_{\mathrm{ddd}}\right)}{x_{\mathrm{dd}}-x_{l}}-\psi _{d,\mathrm{SG},D,1}+\frac{\psi _{\mathrm{fd},\mathrm{SG},D,1}\,\left(x_{\mathrm{ddd}}-x_{l}\right)}{x_{\mathrm{dd}}-x_{l}}\right)}{x_{\mathrm{ddd}}}$
      | Automatically generated on 2025-10-31 19:29:42 .
  State_psi_d_SG_D_1_721af : Inport
  State_psi_gq_SG_D_1_018b7 : Inport  Port=2
  State_psi_kq_SG_D_1_d6793 : Inport  Port=3
  State_psi_q_SG_D_1_b7612 : Inport  Port=4
  State_psi_q_SG_D_1_8370d : Inport  Port=5
  State_psi_1d_SG_D_1_c4246 : Inport  Port=6
  State_psi_d_SG_D_1_20494 : Inport  Port=7
  State_psi_fd_SG_D_1_fa2b7 : Inport  Port=8
  Add_2c987 : Sum
  Add_47f69 : Sum
  Add_5264a : Sum
  Add_86dcf : Sum
  Add_bac03 : Sum
  Add_e4a1b : Sum
  Constant_-1_01ca2 : Constant  Value=-1
  Constant_-1_41c16 : Constant  Value=-1
  Constant_-1_65f4a : Constant  Value=-1
  Constant_-1_6c2b8 : Constant  Value=-1
  Constant_-1_848c8 : Constant  Value=-1
  Constant_x_dd_1628b : Constant  Value=x_dd
  Constant_x_dd_2f324 : Constant  Value=x_dd
  Constant_x_dd_751b3 : Constant  Value=x_dd
  Constant_x_ddd_d5f0d : Constant  Value=x_ddd
  Constant_x_ddd_d6ae6 : Constant  Value=x_ddd
  Constant_x_ddd_fba67 : Constant  Value=x_ddd
  Constant_x_l_0f8d7 : Constant  Value=x_l
  Constant_x_l_801f8 : Constant  Value=x_l
  Constant_x_l_8c956 : Constant  Value=x_l
  Constant_x_l_98c12 : Constant  Value=x_l
  Constant_x_l_c47f6 : Constant  Value=x_l
  Constant_x_l_dbbd4 : Constant  Value=x_l
  Constant_x_qd_878f9 : Constant  Value=x_qd
  Constant_x_qd_9b3d1 : Constant  Value=x_qd
  Constant_x_qd_f6133 : Constant  Value=x_qd
  Constant_x_qdd_4a826 : Constant  Value=x_qdd
  Constant_x_qdd_85457 : Constant  Value=x_qdd
  Constant_x_qdd_b3641 : Constant  Value=x_qdd
  Divide_1595f : Product  Inputs=*/
  Divide_16c19 : Product  Inputs=*/
  Divide_4a09d : Product  Inputs=*/
  Divide_a6ad4 : Product  Inputs=*/
  Divide_e104c : Product  Inputs=*/
  Divide_f0816 : Product  Inputs=*/
  Product_05719 : Product
  Product_0c714 : Product
  Product_3215b : Product
  Product_38a90 : Product
  Product_3abba : Product
  Product_6924e : Product
  Product_7a3e5 : Product
  Product_9d523 : Product
  Product_dd6f6 : Product
  Product_df591 : Product
  Product_e8757 : Product
  Subtract_07918 : Sum  Inputs=+-
  Subtract_2e1dd : Sum  Inputs=+-
  Subtract_56158 : Sum  Inputs=+-
  Subtract_746af : Sum  Inputs=+-
  Subtract_93160 : Sum  Inputs=+-
  Subtract_e4447 : Sum  Inputs=+-
  Subtract_f0ec1 : Sum  Inputs=+-
  Blockout_T_e_SG_D_1_b08e1 : Outport
  wires:
  Product_3215b/1 -> Divide_e104c/1
  Product_7a3e5/1 -> Add_bac03/1
  Divide_e104c/1 -> Subtract_e4447/1
  Constant_-1_01ca2/1 -> Product_7a3e5/1
  Constant_x_l_c47f6/1 -> Product_7a3e5/2
  Constant_x_qdd_b3641/1 -> Add_bac03/2
  Constant_x_qd_9b3d1/1 -> Subtract_2e1dd/1
  Constant_-1_848c8/1 -> Product_e8757/1
  Constant_x_qdd_4a826/1 -> Divide_f0816/2
  Constant_x_qdd_85457/1 -> Subtract_2e1dd/2
  State_psi_q_SG_D_1_8370d/1 -> Product_6924e/1
  Constant_x_dd_1628b/1 -> Subtract_07918/1
  Constant_x_l_0f8d7/1 -> Product_e8757/2
  Subtract_07918/1 -> Product_05719/2
  Constant_-1_6c2b8/1 -> Product_dd6f6/1
  Constant_x_l_dbbd4/1 -> Product_dd6f6/2
  Subtract_f0ec1/1 -> Product_6924e/2
  State_psi_q_SG_D_1_b7612/1 -> Add_86dcf/2
  Constant_-1_65f4a/1 -> Product_df591/1
  State_psi_1d_SG_D_1_c4246/1 -> Product_df591/2
  Constant_x_ddd_fba67/1 -> Subtract_07918/2
  State_psi_gq_SG_D_1_018b7/1 -> Product_3215b/1
  Add_bac03/1 -> Product_3215b/2
  Product_e8757/1 -> Add_e4a1b/1
  Product_0c714/1 -> Product_9d523/1
  Constant_x_qd_878f9/1 -> Add_e4a1b/2
  Product_05719/1 -> Divide_4a09d/1
  State_psi_kq_SG_D_1_d6793/1 -> Product_38a90/1
  Add_e4a1b/1 -> Divide_e104c/2
  Subtract_2e1dd/1 -> Product_38a90/2
  Product_dd6f6/1 -> Add_47f69/1
  Constant_x_qd_f6133/1 -> Add_47f69/2
  Product_38a90/1 -> Divide_a6ad4/1
  Product_df591/1 -> Product_05719/1
  Constant_x_dd_2f324/1 -> Subtract_56158/1
  Constant_x_l_801f8/1 -> Subtract_56158/2
  Constant_x_ddd_d6ae6/1 -> Subtract_93160/1
  Product_6924e/1 -> Divide_16c19/1
  Constant_x_l_8c956/1 -> Subtract_93160/2
  Divide_f0816/1 -> Add_2c987/1
  Product_9d523/1 -> Divide_f0816/1
  Add_47f69/1 -> Divide_a6ad4/2
  Subtract_e4447/1 -> Add_86dcf/1
  Divide_a6ad4/1 -> Subtract_e4447/2
  Subtract_56158/1 -> Divide_4a09d/2
  State_psi_fd_SG_D_1_fa2b7/1 -> Product_3abba/1
  Constant_x_ddd_d5f0d/1 -> Divide_16c19/2
  Subtract_93160/1 -> Product_3abba/2
  Constant_x_dd_751b3/1 -> Subtract_746af/1
  Constant_x_l_98c12/1 -> Subtract_746af/2
  Divide_4a09d/1 -> Add_5264a/1
  Add_5264a/1 -> Subtract_f0ec1/1
  State_psi_d_SG_D_1_20494/1 -> Add_5264a/2
  Product_3abba/1 -> Divide_1595f/1
  Subtract_746af/1 -> Divide_1595f/2
  Constant_-1_41c16/1 -> Product_0c714/1
  State_psi_d_SG_D_1_721af/1 -> Product_0c714/2
  Divide_1595f/1 -> Subtract_f0ec1/2
  Add_86dcf/1 -> Product_9d523/2
  Divide_16c19/1 -> Add_2c987/2
  Add_2c987/1 -> Blockout_T_e_SG_D_1_b08e1/1

== system case8/SG_D_1/d_E_fd_SG_D_1_block ==
  note: d_E_fd_SG_D_1 in case8
      | $\frac{V_{f,\mathrm{SG},D,1}-E_{\mathrm{fd},\mathrm{SG},D,1}\,K_{E}}{T_{E}}$
      | Automatically generated on 2025-10-31 19:29:39 .
  State_E_fd_SG_D_1_e2b7b : Inport
  State_V_f_SG_D_1_1b8c0 : Inport  Port=2
  Add_98939 : Sum
  Constant_-1_6edd9 : Constant  Value=-1
  Constant_K_E_57fca : Constant  Value=K_E
  Constant_T_E_d6f8b : Constant  Value=T_E
  Divide_65d4f : Product  Inputs=*/
  Product_77b09 : Product
  Product_b78fb : Product
  Blockout_d_E_fd_SG_D_1_9b618 : Outport
  wires:
  Add_98939/1 -> Divide_65d4f/1
  Constant_-1_6edd9/1 -> Product_77b09/1
  State_E_fd_SG_D_1_e2b7b/1 -> Product_77b09/2
  Product_77b09/1 -> Product_b78fb/1
  Constant_K_E_57fca/1 -> Product_b78fb/2
  Product_b78fb/1 -> Add_98939/1
  Constant_T_E_d6f8b/1 -> Divide_65d4f/2
  State_V_f_SG_D_1_1b8c0/1 -> Add_98939/2
  Divide_65d4f/1 -> Blockout_d_E_fd_SG_D_1_9b618/1

== system case8/SG_D_1/d_Px_1_SG_D_1_block ==
  note: d_Px_1_SG_D_1 in case8
      | $\frac{w_{\mathrm{SG},D,1}-2\,\pi \,f_{0}}{T_{w}}-\frac{\mathrm{Px}_{1,\mathrm{SG},D,1}}{T_{w}}$
      | Automatically generated on 2025-10-31 19:29:39 .
  State_Px_1_SG_D_1_40f75 : Inport
  State_w_SG_D_1_79126 : Inport  Port=2
  Add_06054 : Sum
  Add_9c6c2 : Sum
  Constant_-1_c8129 : Constant  Value=-1
  Constant_-2.0_b2f8e : Constant  Value=-2.0
  Constant_T_w_48da3 : Constant  Value=T_w
  Constant_T_w_c710b : Constant  Value=T_w
  Constant_f0_78069 : Constant  Value=f0
  Constant_pi_c4842 : Constant  Value=pi
  Divide_94ac3 : Product  Inputs=*/
  Divide_f6ba6 : Product  Inputs=*/
  Product_05999 : Product
  Product_0d846 : Product
  Product_667a0 : Product
  Blockout_d_Px_1_SG_D_1_adb46 : Outport
  wires:
  Add_06054/1 -> Blockout_d_Px_1_SG_D_1_adb46/1
  Constant_-2.0_b2f8e/1 -> Product_05999/1
  Product_0d846/1 -> Divide_f6ba6/1
  State_w_SG_D_1_79126/1 -> Add_9c6c2/2
  Constant_-1_c8129/1 -> Product_0d846/1
  Constant_f0_78069/1 -> Product_667a0/2
  Constant_pi_c4842/1 -> Product_05999/2
  Product_667a0/1 -> Add_9c6c2/1
  Product_05999/1 -> Product_667a0/1
  State_Px_1_SG_D_1_40f75/1 -> Product_0d846/2
  Constant_T_w_c710b/1 -> Divide_f6ba6/2
  Add_9c6c2/1 -> Divide_94ac3/1
  Constant_T_w_48da3/1 -> Divide_94ac3/2
  Divide_f6ba6/1 -> Add_06054/1
  Divide_94ac3/1 -> Add_06054/2

== system case8/SG_D_1/d_Px_2_SG_D_1_block ==
  note: d_Px_2_SG_D_1 in case8
      | $\frac{\mathrm{Px}_{1,\mathrm{SG},D,1}-T_{2}\,\left(\frac{\mathrm{Px}_{1,\mathrm{SG},D,1}}{T_{w}}-\frac{w_{\mathrm{SG},D,1}-2\,\pi \,f_{0}}{T_{w}}\right)}{T_{1}}-\frac{\mathrm{Px}_{2,\mathrm{SG},D,1}}{T_{1}}$
      | Automatically generated on 2025-10-31 19:29:39 .
  State_Px_2_SG_D_1_536b3 : Inport
  State_Px_1_SG_D_1_84ac5 : Inport  Port=2
  State_Px_1_SG_D_1_808d2 : Inport  Port=3
  State_w_SG_D_1_35db8 : Inport  Port=4
  Add_14b7f : Sum
  Add_200ff : Sum
  Add_3fe27 : Sum
  Add_6255e : Sum
  Constant_-1_150f8 : Constant  Value=-1
  Constant_-1_c415b : Constant  Value=-1
  Constant_-2.0_e9300 : Constant  Value=-2.0
  Constant_T_1_49484 : Constant  Value=T_1
  Constant_T_1_6f3c9 : Constant  Value=T_1
  Constant_T_2_f8c80 : Constant  Value=T_2
  Constant_T_w_8f0f4 : Constant  Value=T_w
  Constant_T_w_c5c1c : Constant  Value=T_w
  Constant_f0_b9a76 : Constant  Value=f0
  Constant_pi_1dd6d : Constant  Value=pi
  Divide_0cdc0 : Product  Inputs=*/
  Divide_4a4e1 : Product  Inputs=*/
  Divide_a13a6 : Product  Inputs=*/
  Divide_c1ac9 : Product  Inputs=*/
  Product_085d6 : Product
  Product_129f0 : Product
  Product_25507 : Product
  Product_4816a : Product
  Product_dec3d : Product
  Blockout_d_Px_2_SG_D_1_bf890 : Outport
  wires:
  Constant_-2.0_e9300/1 -> Product_25507/1
  State_w_SG_D_1_35db8/1 -> Add_14b7f/2
  Constant_f0_b9a76/1 -> Product_085d6/2
  Constant_pi_1dd6d/1 -> Product_25507/2
  Add_3fe27/1 -> Product_129f0/2
  Product_085d6/1 -> Add_14b7f/1
  Divide_4a4e1/1 -> Add_3fe27/1
  Product_25507/1 -> Product_085d6/1
  Constant_T_w_c5c1c/1 -> Divide_4a4e1/2
  Constant_-1_c415b/1 -> Product_dec3d/1
  State_Px_1_SG_D_1_808d2/1 -> Product_dec3d/2
  Divide_0cdc0/1 -> Add_200ff/1
  Product_dec3d/1 -> Divide_4a4e1/1
  Add_14b7f/1 -> Divide_a13a6/1
  Constant_T_w_8f0f4/1 -> Divide_a13a6/2
  Divide_a13a6/1 -> Add_3fe27/2
  Constant_T_2_f8c80/1 -> Product_129f0/1
  Constant_-1_150f8/1 -> Product_4816a/1
  State_Px_2_SG_D_1_536b3/1 -> Product_4816a/2
  State_Px_1_SG_D_1_84ac5/1 -> Add_6255e/1
  Product_129f0/1 -> Add_6255e/2
  Add_6255e/1 -> Divide_c1ac9/1
  Product_4816a/1 -> Divide_0cdc0/1
  Constant_T_1_49484/1 -> Divide_0cdc0/2
  Constant_T_1_6f3c9/1 -> Divide_c1ac9/2
  Divide_c1ac9/1 -> Add_200ff/2
  Add_200ff/1 -> Blockout_d_Px_2_SG_D_1_bf890/1

== system case8/SG_D_1/d_Px_3_SG_D_1_block ==
  note: d_Px_3_SG_D_1 in case8
      | $\frac{\mathrm{Px}_{2,\mathrm{SG},D,1}+T_{4}\,\left(\frac{\mathrm{Px}_{1,\mathrm{SG},D,1}-T_{2}\,\left(\frac{\mathrm{Px}_{1,\mathrm{SG},D,1}}{T_{w}}-\frac{w_{\mathrm{SG},D,1}-2\,\pi \,f_{0}}{T_{w}}\right)}{T_{1}}-\frac{\mathrm{Px}_{2,\mathrm{SG},D,1}}{T_{1}}\right)}{T_{3}}-\frac{\mathrm{Px}_{3,\mathrm{SG},D,1}}{T_{3}}$
      | Automatically generated on 2025-10-31 19:29:40 .
  State_Px_3_SG_D_1_97912 : Inport
  State_Px_2_SG_D_1_ec984 : Inport  Port=2
  State_Px_2_SG_D_1_b129a : Inport  Port=3
  State_Px_1_SG_D_1_02f94 : Inport  Port=4
  State_Px_1_SG_D_1_0957c : Inport  Port=5
  State_w_SG_D_1_9ce72 : Inport  Port=6
  Add_06eae : Sum
  Add_2dc8e : Sum
  Add_70a1d : Sum
  Add_abb9b : Sum
  Add_b964f : Sum
  Add_eb275 : Sum
  Constant_-1_6c49c : Constant  Value=-1
  Constant_-1_86ca3 : Constant  Value=-1
  Constant_-1_fc4c7 : Constant  Value=-1
  Constant_-2.0_e93b9 : Constant  Value=-2.0
  Constant_T_1_8c915 : Constant  Value=T_1
  Constant_T_1_969a4 : Constant  Value=T_1
  Constant_T_2_00e84 : Constant  Value=T_2
  Constant_T_3_81e5f : Constant  Value=T_3
  Constant_T_3_ce3df : Constant  Value=T_3
  Constant_T_4_88886 : Constant  Value=T_4
  Constant_T_w_0ff25 : Constant  Value=T_w
  Constant_T_w_7bacf : Constant  Value=T_w
  Constant_f0_cbc32 : Constant  Value=f0
  Constant_pi_2a6fa : Constant  Value=pi
  Divide_37e46 : Product  Inputs=*/
  Divide_9ad44 : Product  Inputs=*/
  Divide_d5877 : Product  Inputs=*/
  Divide_e17f7 : Product  Inputs=*/
  Divide_e87bc : Product  Inputs=*/
  Divide_ec477 : Product  Inputs=*/
  Product_088b7 : Product
  Product_337ad : Product
  Product_6eea2 : Product
  Product_ae96c : Product
  Product_cc383 : Product
  Product_e0253 : Product
  Product_f102c : Product
  Blockout_d_Px_3_SG_D_1_3f1ef : Outport
  wires:
  Constant_T_w_0ff25/1 -> Divide_37e46/2
  Constant_-1_fc4c7/1 -> Product_088b7/1
  Add_eb275/1 -> Blockout_d_Px_3_SG_D_1_3f1ef/1
  Constant_-2.0_e93b9/1 -> Product_cc383/1
  State_w_SG_D_1_9ce72/1 -> Add_b964f/2
  Constant_f0_cbc32/1 -> Product_ae96c/2
  State_Px_1_SG_D_1_0957c/1 -> Product_088b7/2
  Constant_pi_2a6fa/1 -> Product_cc383/2
  Product_ae96c/1 -> Add_b964f/1
  Product_cc383/1 -> Product_ae96c/1
  Product_088b7/1 -> Divide_37e46/1
  Divide_e87bc/1 -> Add_eb275/1
  Constant_T_3_81e5f/1 -> Divide_ec477/2
  Add_b964f/1 -> Divide_e17f7/1
  Constant_T_w_7bacf/1 -> Divide_e17f7/2
  Divide_37e46/1 -> Add_06eae/1
  Divide_e17f7/1 -> Add_06eae/2
  Constant_-1_6c49c/1 -> Product_e0253/1
  Constant_T_2_00e84/1 -> Product_f102c/1
  Add_06eae/1 -> Product_f102c/2
  Constant_-1_86ca3/1 -> Product_6eea2/1
  Divide_ec477/1 -> Add_eb275/2
  Constant_T_3_ce3df/1 -> Divide_e87bc/2
  State_Px_2_SG_D_1_b129a/1 -> Product_6eea2/2
  State_Px_1_SG_D_1_02f94/1 -> Add_70a1d/1
  Divide_9ad44/1 -> Add_2dc8e/1
  Product_f102c/1 -> Add_70a1d/2
  Product_6eea2/1 -> Divide_9ad44/1
  Product_e0253/1 -> Divide_e87bc/1
  Constant_T_1_8c915/1 -> Divide_9ad44/2
  Add_70a1d/1 -> Divide_d5877/1
  Constant_T_1_969a4/1 -> Divide_d5877/2
  Divide_d5877/1 -> Add_2dc8e/2
  Constant_T_4_88886/1 -> Product_337ad/1
  Add_2dc8e/1 -> Product_337ad/2
  State_Px_3_SG_D_1_97912/1 -> Product_e0253/2
  State_Px_2_SG_D_1_ec984/1 -> Add_abb9b/1
  Product_337ad/1 -> Add_abb9b/2
  Add_abb9b/1 -> Divide_ec477/1

== system case8/SG_D_1/d_R_f_SG_D_1_block ==
  note: d_R_f_SG_D_1 in case8
      | $-\frac{R_{f,\mathrm{SG},D,1}-\frac{E_{\mathrm{fd},\mathrm{SG},D,1}\,K_{F}}{T_{F}}}{T_{F}}$
      | Automatically generated on 2025-10-31 19:29:39 .
  State_E_fd_SG_D_1_91fb8 : Inport
  State_R_f_SG_D_1_4464e : Inport  Port=2
  Constant_K_F_38682 : Constant  Value=K_F
  Constant_T_F_48c78 : Constant  Value=T_F
  Constant_T_F_dd612 : Constant  Value=T_F
  Divide_48885 : Product  Inputs=*/
  Divide_e35f5 : Product  Inputs=*/
  Product_aeebb : Product
  Subtract_cbefc : Sum  Inputs=+-
  Blockout_d_R_f_SG_D_1_f74b6 : Outport
  wires:
  Constant_K_F_38682/1 -> Product_aeebb/2
  Product_aeebb/1 -> Divide_48885/1
  State_E_fd_SG_D_1_91fb8/1 -> Product_aeebb/1
  State_R_f_SG_D_1_4464e/1 -> Subtract_cbefc/2
  Constant_T_F_dd612/1 -> Divide_48885/2
  Divide_48885/1 -> Subtract_cbefc/1
  Divide_e35f5/1 -> Blockout_d_R_f_SG_D_1_f74b6/1
  Subtract_cbefc/1 -> Divide_e35f5/1
  Constant_T_F_48c78/1 -> Divide_e35f5/2

== system case8/SG_D_1/d_T_m_SG_D_1_block ==
  note: d_T_m_SG_D_1 in case8
      | $-\frac{T_{m,\mathrm{SG},D,1}-T_{0}+\frac{\mathrm{SpeedPara}\,\left(w_{\mathrm{SG},D,1}-w_{\mathrm{ref}}\right)}{2\,f_{0}\,\pi }}{T_{\mathrm{speed}}}$
      | Automatically generated on 2025-10-31 19:29:36 .
  State_w_SG_D_1_c0f9f : Inport
  State_T_m_SG_D_1_2bf30 : Inport  Port=2
  Add_43d1a : Sum
  Add_5d3af : Sum
  Constant_-1_b0084 : Constant  Value=-1
  Constant_2.0_7cd51 : Constant  Value=2.0
  Constant_SpeedPara_e5c7d : Constant  Value=SpeedPara
  Constant_T_0_12d6c : Constant  Value=T_0
  Constant_T_speed_b9cfd : Constant  Value=T_speed
  Constant_f0_45d49 : Constant  Value=f0
  Constant_pi_e9efc : Constant  Value=pi
  Constant_w_ref_05345 : Constant  Value=w_ref
  Divide_2d322 : Product  Inputs=*/
  Divide_315c4 : Product  Inputs=*/
  Product_3bf98 : Product
  Product_4920f : Product
  Product_af956 : Product
  Product_d5b40 : Product
  Subtract_2b492 : Sum  Inputs=+-
  Blockout_d_T_m_SG_D_1_8754a : Outport
  wires:
  Constant_-1_b0084/1 -> Product_af956/1
  Constant_w_ref_05345/1 -> Add_5d3af/2
  State_w_SG_D_1_c0f9f/1 -> Product_af956/2
  Add_43d1a/1 -> Subtract_2b492/1
  Add_5d3af/1 -> Product_4920f/2
  Product_af956/1 -> Add_5d3af/1
  Constant_2.0_7cd51/1 -> Product_d5b40/1
  Constant_pi_e9efc/1 -> Product_d5b40/2
  Constant_SpeedPara_e5c7d/1 -> Product_4920f/1
  Product_d5b40/1 -> Product_3bf98/1
  Constant_f0_45d49/1 -> Product_3bf98/2
  Constant_T_speed_b9cfd/1 -> Divide_2d322/2
  Product_4920f/1 -> Divide_315c4/1
  Product_3bf98/1 -> Divide_315c4/2
  Divide_315c4/1 -> Add_43d1a/1
  Constant_T_0_12d6c/1 -> Add_43d1a/2
  State_T_m_SG_D_1_2bf30/1 -> Subtract_2b492/2
  Subtract_2b492/1 -> Divide_2d322/1
  Divide_2d322/1 -> Blockout_d_T_m_SG_D_1_8754a/1
